simulink model "constant_f_V_PWM"  (R2016a)
settings: Solver=FixedStepAuto  StartTime=0.0  StopTime=3  FixedStep=0.00003  RelTol=1e-3
undefined symbols (not defined in the file): Lm, Lr, Ls, M_ab02abc, M_abc2ab0, Rr, sig
libraries: powerlib_meascontrol x2, simulink x1
settings Model: Creator=ebenera  LastModifiedBy=ebenera

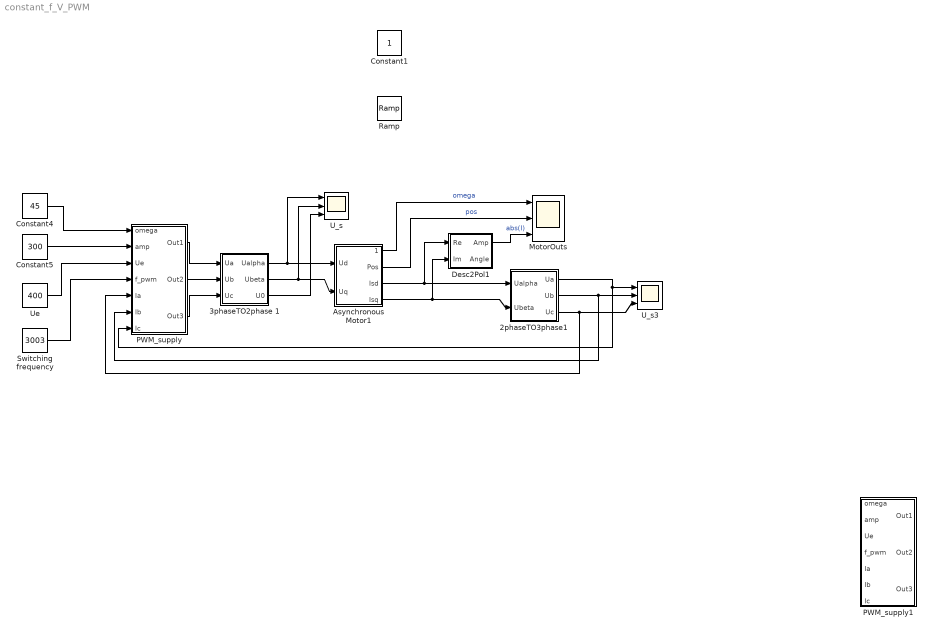
== system constant_f_V_PWM ==
  2phaseTO3phase1 : Subsystem
  3phaseTO2phase 1 : Subsystem
  Asynchronous Motor1 : Subsystem
  Constant4 : Constant  Value=45
  Constant5 : Constant  Value=300
  Desc2Pol1 : Subsystem
  MotorOuts : Scope  NumInputPorts=3
  PWM_supply : Subsystem
  PWM_supply1 : Subsystem
  Switching frequency : Constant  Value=3003
  U_s : Scope  NumInputPorts=3
  U_s3 : Scope  NumInputPorts=3
  Ue : Constant  Value=400
  " " : Constant  IOType=siggen
  Constant1 : Constant  IOType=siggen
  Ramp : simulink/Sources/Ramp  IOType=siggen  slope=1  start=0  X0=0
  wires:
  Asynchronous Motor1/4(Isq) -> 2phaseTO3phase1/2(Ubeta), Desc2Pol1/2(Im)
  Asynchronous Motor1/3(Isd) -> 2phaseTO3phase1/1(Ualpha), Desc2Pol1/1(Re)
  2phaseTO3phase1/1(Ua) -> U_s3/1, PWM_supply/7(Ic)
  2phaseTO3phase1/2(Ub) -> U_s3/2, PWM_supply/6(Ib)
  2phaseTO3phase1/3(Uc) -> U_s3/3, PWM_supply/5(Ia)
  3phaseTO2phase 1/1(Ualpha) -> U_s/1, Asynchronous Motor1/1(Ud)
  3phaseTO2phase 1/2(Ubeta) -> Asynchronous Motor1/2(Uq), U_s/2
  3phaseTO2phase 1/3(U0) -> U_s/3
  Desc2Pol1/1(Amp) -> MotorOuts/3  "abs(I)"
  Asynchronous Motor1/1(Omega) -> MotorOuts/1  "omega"
  Asynchronous Motor1/2(Pos) -> MotorOuts/2  "pos"
  Constant4/1 -> PWM_supply/1(omega)
  Constant5/1 -> PWM_supply/2(amp)
  Ue/1 -> PWM_supply/3(Ue)
  Switching frequency/1 -> PWM_supply/4(f_pwm)
  PWM_supply/1(Out1) -> 3phaseTO2phase 1/1(Ua)
  PWM_supply/2(Out2) -> 3phaseTO2phase 1/2(Ub)
  PWM_supply/3(Out3) -> 3phaseTO2phase 1/3(Uc)

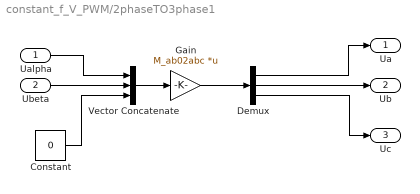
== system constant_f_V_PWM/2phaseTO3phase1 ==
  Ualpha : Inport
  Ubeta : Inport  Port=2
  Constant : Constant  Value=0
  Demux : Demux  Outputs=3
  Gain : Gain  Gain=M_ab02abc  Multiplication=Matrix(K*u)
  Vector Concatenate : Concatenate  NumInputs=3
  Ua : Outport
  Ub : Outport  Port=2
  Uc : Outport  Port=3
  wires:
  Vector Concatenate/1 -> Gain/1
  Ualpha/1 -> Vector Concatenate/1
  Demux/3 -> Uc/1
  Gain/1 -> Demux/1
  Constant/1 -> Vector Concatenate/3
  Ubeta/1 -> Vector Concatenate/2
  Demux/1 -> Ua/1
  Demux/2 -> Ub/1

== system constant_f_V_PWM/3phaseTO2phase 1 ==
  Ua : Inport
  Ub : Inport  Port=2
  Uc : Inport  Port=3
  Demux : Demux  Outputs=3
  Gain : Gain  Gain=M_abc2ab0  Multiplication=Matrix(K*u)
  Vector Concatenate : Concatenate  NumInputs=3
  Ualpha : Outport
  Ubeta : Outport  Port=2
  U0 : Outport  Port=3
  wires:
  Vector Concatenate/1 -> Gain/1
  Ua/1 -> Vector Concatenate/1
  Demux/3 -> U0/1
  Gain/1 -> Demux/1
  Uc/1 -> Vector Concatenate/3
  Ub/1 -> Vector Concatenate/2
  Demux/1 -> Ualpha/1
  Demux/2 -> Ubeta/1

== system constant_f_V_PWM/Asynchronous Motor1 ==
  Ud : Inport
  Uq : Inport  Port=2
  MeasAsync : Scope  NumInputPorts=3
  Motor Electric : Subsystem
  Motor mechanic : Subsystem
  Omega : Outport
  Pos : Outport  Port=2
  Isd : Outport  Port=3
  Isq : Outport  Port=4
  wires:
  Motor mechanic/2(Pos) -> MeasAsync/3, Pos/1  "Pos"
  Motor mechanic/1(Omega) -> Motor Electric/3(Omega), Omega/1, MeasAsync/2  "OMEGA"
  Motor Electric/1(Me) -> MeasAsync/1, Motor mechanic/1("Torq ")  "Torq"
  Motor Electric/2(Isd) -> Isd/1
  Motor Electric/3(Isq) -> Isq/1
  Uq/1 -> Motor Electric/2(Uq)
  Ud/1 -> Motor Electric/1(Ud)

== system constant_f_V_PWM/Desc2Pol1 ==
  Re : Inport
  Im : Inport  Port=2
  Complex to Magnitude-Angle2 : ComplexToMagnitudeAngle
  Real-Imag to Complex3 : RealImagToComplex
  Amp : Outport
  Angle : Outport  Port=2
  wires:
  Complex to Magnitude-Angle2/1 -> Amp/1
  Real-Imag to Complex3/1 -> Complex to Magnitude-Angle2/1
  Complex to Magnitude-Angle2/2 -> Angle/1
  Re/1 -> Real-Imag to Complex3/1
  Im/1 -> Real-Imag to Complex3/2

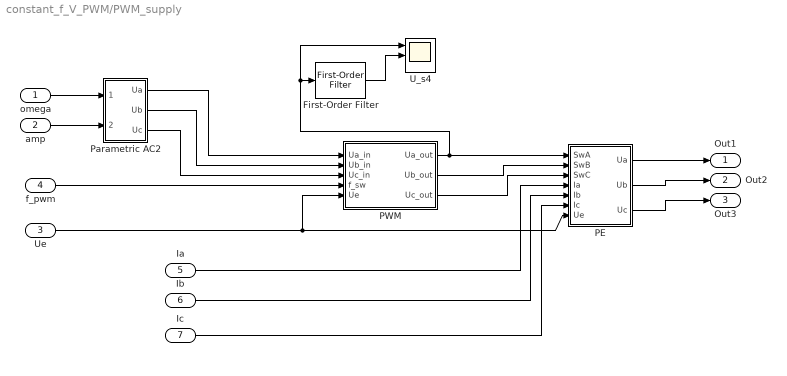
== system constant_f_V_PWM/PWM_supply ==
  omega : Inport
  amp : Inport  Port=2
  Ue : Inport  Port=3
  f_pwm : Inport  Port=4
  Ia : Inport  Port=5
  Ib : Inport  Port=6
  Ic : Inport  Port=7
  First-Order Filter : powerlib_meascontrol/Filters/First-Order Filter  FilterType=Lowpass  Tc=1/400  Ts=0  Initialize=on  Vac_Init=[0, 0, 60]  Vdc_Init=0  PlotResponse=off  FreqRange="[0,  200,  1]"
  PE : Subsystem
  PWM : Subsystem
  Parametric AC2 : Subsystem  Description=Generates a 3 phase supply with the given angular speed, and aplitude.
  U_s4 : Scope  NumInputPorts=3
  Out1 : Outport
  Out2 : Outport  Port=2
  Out3 : Outport  Port=3
  wires:
  Ic/1 -> PE/6(Ic)
  Ia/1 -> PE/4(Ia)
  Ib/1 -> PE/5(Ib)
  Parametric AC2/3(Uc) -> PWM/3(Uc_in)
  f_pwm/1 -> PWM/4(f_sw)
  Parametric AC2/2(Ub) -> PWM/2(Ub_in)
  amp/1 -> Parametric AC2/2(Amp)
  First-Order Filter/1 -> U_s4/2
  PWM/2(Ub_out) -> PE/2(SwB)
  PWM/1(Ua_out) -> PE/1(SwA), U_s4/1, First-Order Filter/1
  PWM/3(Uc_out) -> PE/3(SwC)
  omega/1 -> Parametric AC2/1(Omega)
  Parametric AC2/1(Ua) -> PWM/1(Ua_in)
  PE/1(Ua) -> Out1/1
  PE/2(Ub) -> Out2/1
  PE/3(Uc) -> Out3/1
  Ue/1 -> PE/7(Ue), PWM/5(Ue)

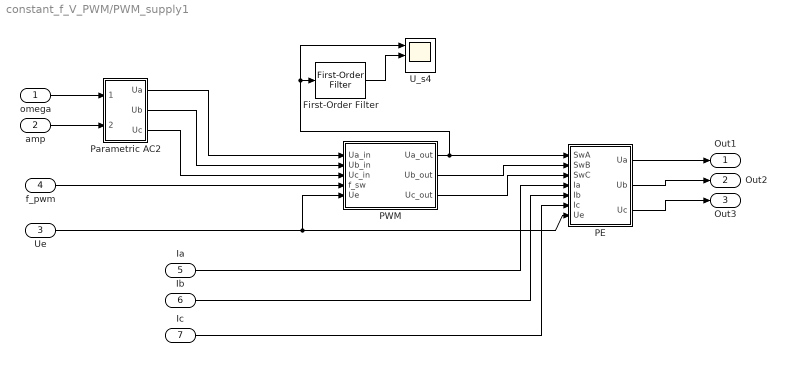
== system constant_f_V_PWM/PWM_supply1 ==
  omega : Inport
  amp : Inport  Port=2
  Ue : Inport  Port=3
  f_pwm : Inport  Port=4
  Ia : Inport  Port=5
  Ib : Inport  Port=6
  Ic : Inport  Port=7
  First-Order Filter : powerlib_meascontrol/Filters/First-Order Filter  FilterType=Lowpass  Tc=1/400  Ts=0  Initialize=on  Vac_Init=[0, 0, 60]  Vdc_Init=0  PlotResponse=off  FreqRange="[0,  200,  1]"
  PE : Subsystem
  PWM : Subsystem
  Parametric AC2 : Subsystem  Description=Generates a 3 phase supply with the given angular speed, and aplitude.
  U_s4 : Scope  NumInputPorts=3
  Out1 : Outport
  Out2 : Outport  Port=2
  Out3 : Outport  Port=3
  wires:
  Ic/1 -> PE/6(Ic)
  Ia/1 -> PE/4(Ia)
  Ib/1 -> PE/5(Ib)
  Parametric AC2/3(Uc) -> PWM/3(Uc_in)
  f_pwm/1 -> PWM/4(f_sw)
  Parametric AC2/2(Ub) -> PWM/2(Ub_in)
  amp/1 -> Parametric AC2/2(Amp)
  First-Order Filter/1 -> U_s4/2
  PWM/2(Ub_out) -> PE/2(SwB)
  PWM/1(Ua_out) -> PE/1(SwA), U_s4/1, First-Order Filter/1
  PWM/3(Uc_out) -> PE/3(SwC)
  omega/1 -> Parametric AC2/1(Omega)
  Parametric AC2/1(Ua) -> PWM/1(Ua_in)
  PE/1(Ua) -> Out1/1
  PE/2(Ub) -> Out2/1
  PE/3(Uc) -> Out3/1
  Ue/1 -> PE/7(Ue), PWM/5(Ue)

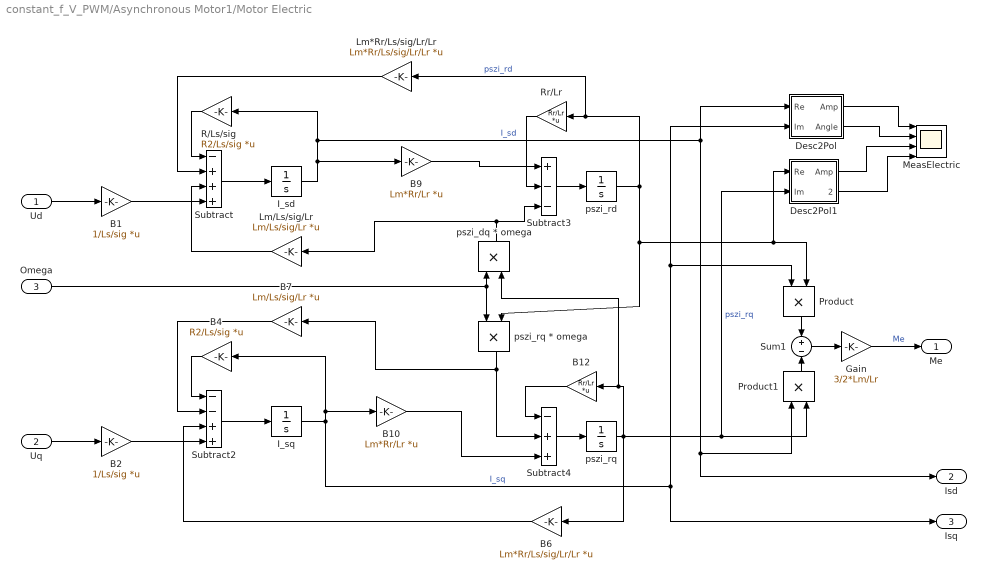
== system constant_f_V_PWM/Asynchronous Motor1/Motor Electric ==
  Ud : Inport
  Uq : Inport  Port=2
  Omega : Inport  Port=3
  B1 : Gain  Gain=1/Ls/sig  Multiplication=Matrix(K*u)
  B10 : Gain  Gain=Lm*Rr/Lr  Multiplication=Matrix(K*u)
  B12 : Gain  Gain=Rr/Lr  Multiplication=Matrix(K*u)
  B2 : Gain  Gain=1/Ls/sig  Multiplication=Matrix(K*u)
  B4 : Gain  Gain=R2/Ls/sig  Multiplication=Matrix(K*u)
  B6 : Gain  Gain=Lm*Rr/Ls/sig/Lr/Lr  Multiplication=Matrix(K*u)
  B7 : Gain  Gain=Lm/Ls/sig/Lr  Multiplication=Matrix(K*u)
  B9 : Gain  Gain=Lm*Rr/Lr  Multiplication=Matrix(K*u)
  Desc2Pol : Subsystem
  Desc2Pol1 : Subsystem
  Gain : Gain  Gain=3/2*Lm/Lr
  I_sd : Integrator
  I_sq : Integrator
  Lm*Rr/Ls/sig/Lr/Lr : Gain  Gain=Lm*Rr/Ls/sig/Lr/Lr  Multiplication=Matrix(K*u)
  Lm/Ls/sig/Lr : Gain  Gain=Lm/Ls/sig/Lr  Multiplication=Matrix(K*u)
  MeasElectric : Scope  NumInputPorts=4
  Product : Product
  Product1 : Product
  R/Ls/sig : Gain  Gain=R2/Ls/sig  Multiplication=Matrix(K*u)
  Rr/Lr : Gain  Gain=Rr/Lr  Multiplication=Matrix(K*u)
  Subtract : Sum  Inputs=-+++
  Subtract2 : Sum  Inputs=--++
  Subtract3 : Sum  Inputs=+--
  Subtract4 : Sum  Inputs=-++
  Sum1 : Sum  Inputs=+-
  pszi_dq * omega : Product
  pszi_rd : Integrator
  "pszi_rq " : Integrator
  pszi_rq * omega : Product
  Me : Outport
  Isd : Outport  Port=2
  Isq : Outport  Port=3
  wires:
  pszi_rq * omega/1 -> Subtract4/2, B7/1
  Subtract/1 -> I_sd/1
  B12/1 -> Subtract4/1
  Product1/1 -> Sum1/2
  Lm*Rr/Ls/sig/Lr/Lr/1 -> Subtract/2
  Product/1 -> Sum1/1
  I_sq/1 -> Product/1, Desc2Pol/2(Im), Isq/1, B10/1, B4/1  "I_sq"
  I_sd/1 -> B9/1, Isd/1, Product1/1, Desc2Pol/1(Re), R/Ls/sig/1  "I_sd"
  Sum1/1 -> Gain/1
  R/Ls/sig/1 -> Subtract/1
  B6/1 -> Subtract2/3
  B4/1 -> Subtract2/1
  pszi_dq * omega/1 -> Subtract3/3, Lm/Ls/sig/Lr/1
  Omega/1 -> pszi_rq * omega/1, pszi_dq * omega/1
  B9/1 -> Subtract3/1
  Rr/Lr/1 -> Subtract3/2
  pszi_rd/1 -> Product/2, Desc2Pol1/1(Re), pszi_rq * omega/2, Lm*Rr/Ls/sig/Lr/Lr/1, Rr/Lr/1  "pszi_rd"
  Lm/Ls/sig/Lr/1 -> Subtract/3
  "pszi_rq "/1 -> B6/1, Product1/2, Desc2Pol1/2(Im), pszi_dq * omega/2, B12/1  "pszi_rq"
  B7/1 -> Subtract2/2
  Gain/1 -> Me/1  "Me"
  B10/1 -> Subtract4/3
  Subtract4/1 -> "pszi_rq "/1
  Subtract2/1 -> I_sq/1
  Subtract3/1 -> pszi_rd/1
  Uq/1 -> B2/1
  Ud/1 -> B1/1
  B1/1 -> Subtract/4
  B2/1 -> Subtract2/4
  Desc2Pol/1(Amp) -> MeasElectric/1
  Desc2Pol/2(Angle) -> MeasElectric/2
  Desc2Pol1/1(Amp) -> MeasElectric/3
  Desc2Pol1/2(Angle) -> MeasElectric/4

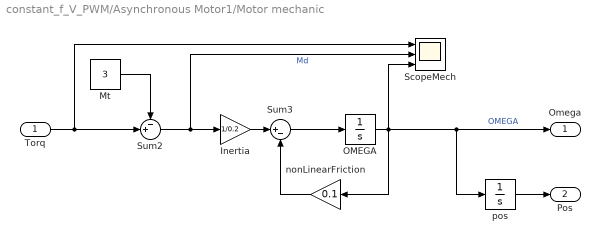
== system constant_f_V_PWM/Asynchronous Motor1/Motor mechanic ==
  "Torq " : Inport
  Inertia : Gain  Gain=1/0.2
  Mt : Constant  Value=3
  OMEGA : Integrator
  ScopeMech : Scope  NumInputPorts=3
  Sum2 : Sum  Inputs=-+|
  Sum3 : Sum  Inputs=|+-
  nonLinearFriction : Gain  Gain=0.1
  pos : Integrator  WrapState=on
  Omega : Outport
  Pos : Outport  Port=2
  wires:
  "Torq "/1 -> ScopeMech/1, Sum2/2
  OMEGA/1 -> ScopeMech/3, pos/1, Omega/1, nonLinearFriction/1  "OMEGA"
  Sum3/1 -> OMEGA/1
  Sum2/1 -> Inertia/1, ScopeMech/2  "Md"
  Mt/1 -> Sum2/1
  nonLinearFriction/1 -> Sum3/2
  Inertia/1 -> Sum3/1
  pos/1 -> Pos/1

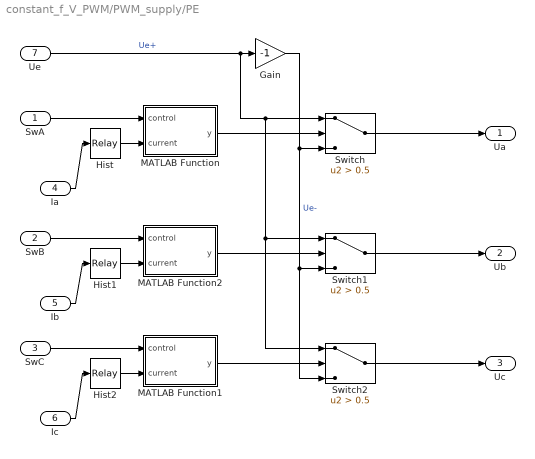
== system constant_f_V_PWM/PWM_supply/PE ==
  SwA : Inport
  SwB : Inport  Port=2
  SwC : Inport  Port=3
  Ia : Inport  Port=4
  Ib : Inport  Port=5
  Ic : Inport  Port=6
  Ue : Inport  Port=7
  Gain : Gain  Gain=-1
  Hist : Relay  OnSwitchValue=0.1  OffSwitchValue=-0.1  OffOutputValue=-1
  Hist1 : Relay  OnSwitchValue=0.1  OffSwitchValue=-0.1  OffOutputValue=-1
  Hist2 : Relay  OnSwitchValue=0.1  OffSwitchValue=-0.1  OffOutputValue=-1
  MATLAB Function : MATLAB Function  TreatAsAtomicUnit=on
  MATLAB Function1 : MATLAB Function  TreatAsAtomicUnit=on
  MATLAB Function2 : MATLAB Function  TreatAsAtomicUnit=on
  Switch : Switch  Criteria=u2 > Threshold  Threshold=0.5
  Switch1 : Switch  Criteria=u2 > Threshold  Threshold=0.5
  Switch2 : Switch  Criteria=u2 > Threshold  Threshold=0.5
  Ua : Outport
  Ub : Outport  Port=2
  Uc : Outport  Port=3
  wires:
  Gain/1 -> Switch2/3, Switch1/3, Switch/3  "Ue-"
  Switch/1 -> Ua/1
  Ue/1 -> Switch/1, Switch1/1, Switch2/1, Gain/1  "Ue+"
  Switch1/1 -> Ub/1
  Switch2/1 -> Uc/1
  MATLAB Function/1(y) -> Switch/2
  MATLAB Function2/1(y) -> Switch1/2
  MATLAB Function1/1(y) -> Switch2/2
  SwB/1 -> MATLAB Function2/1(control)
  SwA/1 -> MATLAB Function/1(control)
  SwC/1 -> MATLAB Function1/1(control)
  Ia/1 -> Hist/1
  Hist/1 -> MATLAB Function/2(current)
  Ib/1 -> Hist1/1
  Hist1/1 -> MATLAB Function2/2(current)
  Hist2/1 -> MATLAB Function1/2(current)
  Ic/1 -> Hist2/1

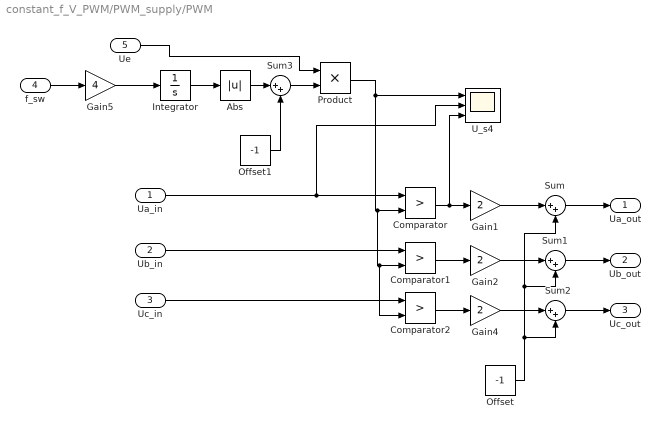
== system constant_f_V_PWM/PWM_supply/PWM ==
  Ua_in : Inport
  Ub_in : Inport  Port=2
  Uc_in : Inport  Port=3
  f_sw : Inport  Port=4
  Ue : Inport  Port=5
  Abs : Abs
  Comparator : RelationalOperator  Operator=>  OutDataTypeStr=boolean
  Comparator1 : RelationalOperator  Operator=>  OutDataTypeStr=boolean
  Comparator2 : RelationalOperator  Operator=>  OutDataTypeStr=boolean
  Gain1 : Gain  Gain=2
  Gain2 : Gain  Gain=2
  Gain4 : Gain  Gain=2
  Gain5 : Gain  Gain=4
  Integrator : Integrator  WrapState=on  WrappedStateUpperValue=2  WrappedStateLowerValue=-2
  Offset : Constant  Value=-1
  Offset1 : Constant  Value=-1
  Product : Product
  Sum{,1..3} (4 alike) : Sum  Inputs=|++
  U_s4 : Scope  NumInputPorts=3
  Ua_out : Outport
  Ub_out : Outport  Port=2
  Uc_out : Outport  Port=3
  wires:
  Uc_in/1 -> Comparator2/1
  Ub_in/1 -> Comparator1/1
  Ua_in/1 -> U_s4/2, Comparator/1
  Comparator/1 -> Gain1/1, U_s4/3
  Product/1 -> U_s4/1, Comparator2/2, Comparator1/2, Comparator/2
  Gain2/1 -> Sum1/1
  Comparator1/1 -> Gain2/1
  Comparator2/1 -> Gain4/1
  Gain4/1 -> Sum2/1
  Sum2/1 -> Uc_out/1
  Sum1/1 -> Ub_out/1
  Sum/1 -> Ua_out/1
  Gain1/1 -> Sum/1
  Offset/1 -> Sum2/2, Sum1/2, Sum/2
  Gain5/1 -> Integrator/1
  f_sw/1 -> Gain5/1
  Ue/1 -> Product/1
  Integrator/1 -> Abs/1
  Offset1/1 -> Sum3/2
  Abs/1 -> Sum3/1
  Sum3/1 -> Product/2

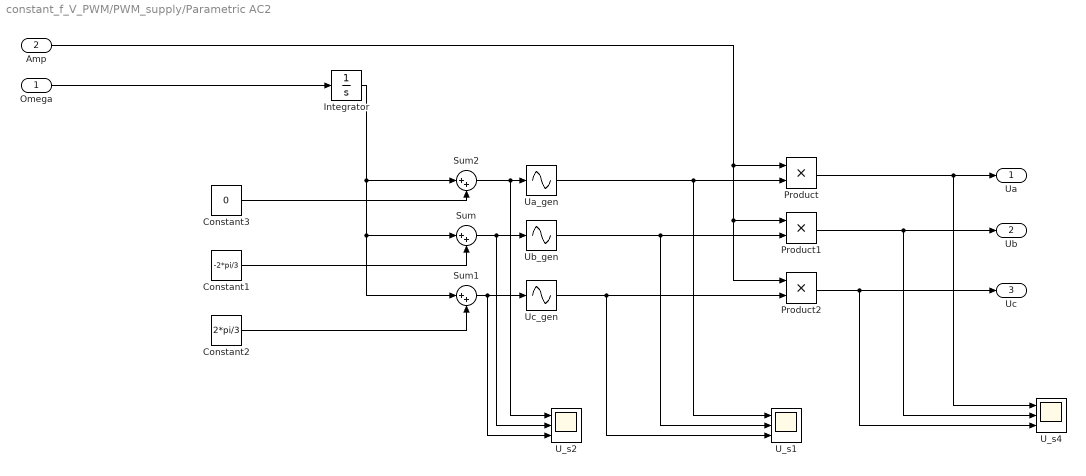
== system constant_f_V_PWM/PWM_supply/Parametric AC2 ==
  Omega : Inport
  Amp : Inport  Port=2
  Constant1 : Constant  Value=-2*pi/3
  Constant2 : Constant  Value=2*pi/3
  Constant3 : Constant  Value=0
  Integrator : Integrator  WrapState=on
  Product : Product
  Product1 : Product
  Product2 : Product
  Sum : Sum  Inputs=|++
  Sum1 : Sum  Inputs=|++
  Sum2 : Sum  Inputs=|++
  U_s1 : Scope  NumInputPorts=3
  U_s2 : Scope  NumInputPorts=3
  U_s4 : Scope  NumInputPorts=3
  Ua_gen : Sin  TimeSource=Use external signal  SampleTime=0
  Ub_gen : Sin  TimeSource=Use external signal  SampleTime=0
  Uc_gen : Sin  TimeSource=Use external signal  SampleTime=0
  Ua : Outport
  Ub : Outport  Port=2
  Uc : Outport  Port=3
  wires:
  Sum/1 -> U_s2/2, Ub_gen/1
  Omega/1 -> Integrator/1
  Constant1/1 -> Sum/2
  Constant2/1 -> Sum1/2
  Sum1/1 -> U_s2/3, Uc_gen/1
  Sum2/1 -> U_s2/1, Ua_gen/1
  Constant3/1 -> Sum2/2
  Integrator/1 -> Sum2/1, Sum1/1, Sum/1
  Product/1 -> U_s4/1, Ua/1
  Product2/1 -> U_s4/3, Uc/1
  Product1/1 -> U_s4/2, Ub/1
  Amp/1 -> Product/1, Product1/1, Product2/1
  Ua_gen/1 -> U_s1/1, Product/2
  Uc_gen/1 -> U_s1/3, Product2/2
  Ub_gen/1 -> U_s1/2, Product1/2

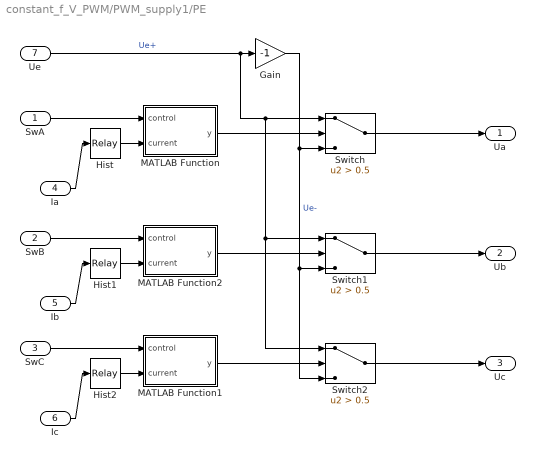
== system constant_f_V_PWM/PWM_supply1/PE ==
  SwA : Inport
  SwB : Inport  Port=2
  SwC : Inport  Port=3
  Ia : Inport  Port=4
  Ib : Inport  Port=5
  Ic : Inport  Port=6
  Ue : Inport  Port=7
  Gain : Gain  Gain=-1
  Hist : Relay  OnSwitchValue=0.1  OffSwitchValue=-0.1  OffOutputValue=-1
  Hist1 : Relay  OnSwitchValue=0.1  OffSwitchValue=-0.1  OffOutputValue=-1
  Hist2 : Relay  OnSwitchValue=0.1  OffSwitchValue=-0.1  OffOutputValue=-1
  MATLAB Function : MATLAB Function  TreatAsAtomicUnit=on
  MATLAB Function1 : MATLAB Function  TreatAsAtomicUnit=on
  MATLAB Function2 : MATLAB Function  TreatAsAtomicUnit=on
  Switch : Switch  Criteria=u2 > Threshold  Threshold=0.5
  Switch1 : Switch  Criteria=u2 > Threshold  Threshold=0.5
  Switch2 : Switch  Criteria=u2 > Threshold  Threshold=0.5
  Ua : Outport
  Ub : Outport  Port=2
  Uc : Outport  Port=3
  wires:
  Gain/1 -> Switch2/3, Switch1/3, Switch/3  "Ue-"
  Switch/1 -> Ua/1
  Ue/1 -> Switch/1, Switch1/1, Switch2/1, Gain/1  "Ue+"
  Switch1/1 -> Ub/1
  Switch2/1 -> Uc/1
  MATLAB Function/1(y) -> Switch/2
  MATLAB Function2/1(y) -> Switch1/2
  MATLAB Function1/1(y) -> Switch2/2
  SwB/1 -> MATLAB Function2/1(control)
  SwA/1 -> MATLAB Function/1(control)
  SwC/1 -> MATLAB Function1/1(control)
  Ia/1 -> Hist/1
  Hist/1 -> MATLAB Function/2(current)
  Ib/1 -> Hist1/1
  Hist1/1 -> MATLAB Function2/2(current)
  Hist2/1 -> MATLAB Function1/2(current)
  Ic/1 -> Hist2/1

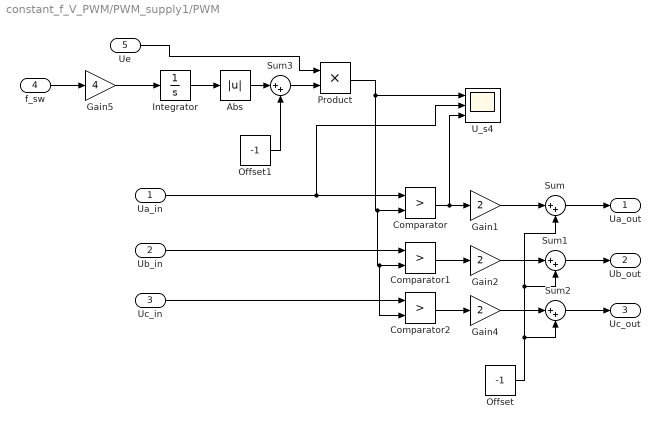
== system constant_f_V_PWM/PWM_supply1/PWM ==
  Ua_in : Inport
  Ub_in : Inport  Port=2
  Uc_in : Inport  Port=3
  f_sw : Inport  Port=4
  Ue : Inport  Port=5
  Abs : Abs
  Comparator : RelationalOperator  Operator=>  OutDataTypeStr=boolean
  Comparator1 : RelationalOperator  Operator=>  OutDataTypeStr=boolean
  Comparator2 : RelationalOperator  Operator=>  OutDataTypeStr=boolean
  Gain1 : Gain  Gain=2
  Gain2 : Gain  Gain=2
  Gain4 : Gain  Gain=2
  Gain5 : Gain  Gain=4
  Integrator : Integrator  WrapState=on  WrappedStateUpperValue=2  WrappedStateLowerValue=-2
  Offset : Constant  Value=-1
  Offset1 : Constant  Value=-1
  Product : Product
  Sum{,1..3} (4 alike) : Sum  Inputs=|++
  U_s4 : Scope  NumInputPorts=3
  Ua_out : Outport
  Ub_out : Outport  Port=2
  Uc_out : Outport  Port=3
  wires:
  Uc_in/1 -> Comparator2/1
  Ub_in/1 -> Comparator1/1
  Ua_in/1 -> U_s4/2, Comparator/1
  Comparator/1 -> Gain1/1, U_s4/3
  Product/1 -> U_s4/1, Comparator2/2, Comparator1/2, Comparator/2
  Gain2/1 -> Sum1/1
  Comparator1/1 -> Gain2/1
  Comparator2/1 -> Gain4/1
  Gain4/1 -> Sum2/1
  Sum2/1 -> Uc_out/1
  Sum1/1 -> Ub_out/1
  Sum/1 -> Ua_out/1
  Gain1/1 -> Sum/1
  Offset/1 -> Sum2/2, Sum1/2, Sum/2
  Gain5/1 -> Integrator/1
  f_sw/1 -> Gain5/1
  Ue/1 -> Product/1
  Integrator/1 -> Abs/1
  Offset1/1 -> Sum3/2
  Abs/1 -> Sum3/1
  Sum3/1 -> Product/2

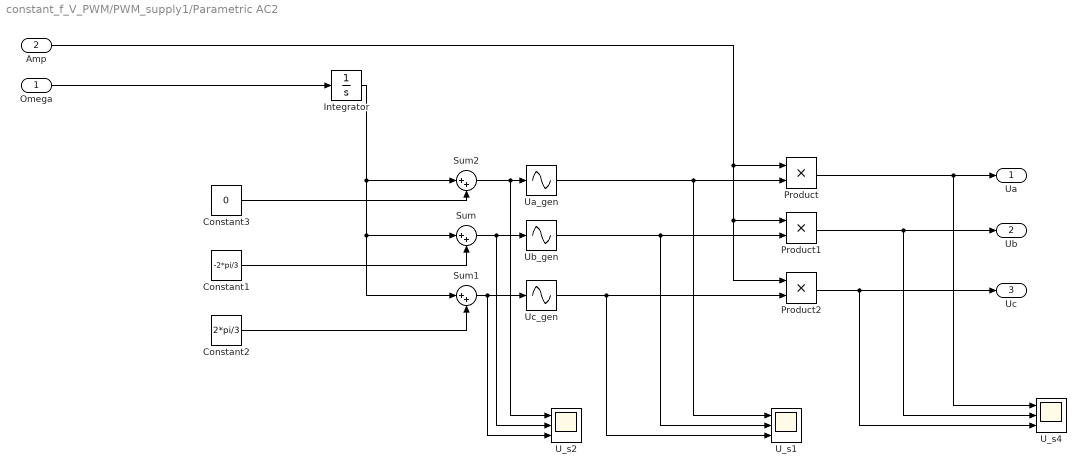
== system constant_f_V_PWM/PWM_supply1/Parametric AC2 ==
  Omega : Inport
  Amp : Inport  Port=2
  Constant1 : Constant  Value=-2*pi/3
  Constant2 : Constant  Value=2*pi/3
  Constant3 : Constant  Value=0
  Integrator : Integrator  WrapState=on
  Product : Product
  Product1 : Product
  Product2 : Product
  Sum : Sum  Inputs=|++
  Sum1 : Sum  Inputs=|++
  Sum2 : Sum  Inputs=|++
  U_s1 : Scope  NumInputPorts=3
  U_s2 : Scope  NumInputPorts=3
  U_s4 : Scope  NumInputPorts=3
  Ua_gen : Sin  TimeSource=Use external signal  SampleTime=0
  Ub_gen : Sin  TimeSource=Use external signal  SampleTime=0
  Uc_gen : Sin  TimeSource=Use external signal  SampleTime=0
  Ua : Outport
  Ub : Outport  Port=2
  Uc : Outport  Port=3
  wires:
  Sum/1 -> U_s2/2, Ub_gen/1
  Omega/1 -> Integrator/1
  Constant1/1 -> Sum/2
  Constant2/1 -> Sum1/2
  Sum1/1 -> U_s2/3, Uc_gen/1
  Sum2/1 -> U_s2/1, Ua_gen/1
  Constant3/1 -> Sum2/2
  Integrator/1 -> Sum2/1, Sum1/1, Sum/1
  Product/1 -> U_s4/1, Ua/1
  Product2/1 -> U_s4/3, Uc/1
  Product1/1 -> U_s4/2, Ub/1
  Amp/1 -> Product/1, Product1/1, Product2/1
  Ua_gen/1 -> U_s1/1, Product/2
  Uc_gen/1 -> U_s1/3, Product2/2
  Ub_gen/1 -> U_s1/2, Product1/2

== system constant_f_V_PWM/Asynchronous Motor1/Motor Electric/Desc2Pol ==
  Re : Inport
  Im : Inport  Port=2
  Complex to Magnitude-Angle2 : ComplexToMagnitudeAngle
  Real-Imag to Complex3 : RealImagToComplex
  Amp : Outport
  Angle : Outport  Port=2
  wires:
  Complex to Magnitude-Angle2/1 -> Amp/1
  Real-Imag to Complex3/1 -> Complex to Magnitude-Angle2/1
  Complex to Magnitude-Angle2/2 -> Angle/1
  Re/1 -> Real-Imag to Complex3/1
  Im/1 -> Real-Imag to Complex3/2

== system constant_f_V_PWM/Asynchronous Motor1/Motor Electric/Desc2Pol1 ==
  Re : Inport
  Im : Inport  Port=2
  Complex to Magnitude-Angle2 : ComplexToMagnitudeAngle
  Real-Imag to Complex3 : RealImagToComplex
  Amp : Outport
  Angle : Outport  Port=2
  wires:
  Complex to Magnitude-Angle2/1 -> Amp/1
  Real-Imag to Complex3/1 -> Complex to Magnitude-Angle2/1
  Complex to Magnitude-Angle2/2 -> Angle/1
  Re/1 -> Real-Imag to Complex3/1
  Im/1 -> Real-Imag to Complex3/2

== matlab function constant_f_V_PWM/PWM_supply/PE/MATLAB Function1 ==
  data: control input; y output; current input
function y = fcn(control, current)
	if control >= 1
        y = 1;
    elseif control <= -1
        y=-1;
    elseif(current>0)
        y = -1;
    else
        y = 1;
    end
end

== matlab function constant_f_V_PWM/PWM_supply/PE/MATLAB Function ==
  data: control input; y output; current input
function y = fcn(control, current)
	if control > 0.5
        y = 1;
    elseif control < -0.5
        y=-1;
    elseif(current>0)
        y = -1;
    else
        y = 1;
    end
end

== matlab function constant_f_V_PWM/PWM_supply/PE/MATLAB Function2 ==
  data: control input; y output; current input
function y = fcn(control, current)
	if control >= 1
        y = 1;
    elseif control <= -1
        y=-1;
    elseif(current>0)
        y = -1;
    else
        y = 1;
    end
end

== matlab function constant_f_V_PWM/PWM_supply1/PE/MATLAB Function ==
  data: control input; y output; current input
function y = fcn(control, current)
	if control > 0.5
        y = 1;
    elseif control < -0.5
        y=-1;
    elseif(current>0)
        y = -1;
    else
        y = 1;
    end
end

== matlab function constant_f_V_PWM/PWM_supply1/PE/MATLAB Function1 ==
  data: control input; y output; current input
function y = fcn(control, current)
	if control >= 1
        y = 1;
    elseif control <= -1
        y=-1;
    elseif(current>0)
        y = -1;
    else
        y = 1;
    end
end

== matlab function constant_f_V_PWM/PWM_supply1/PE/MATLAB Function2 ==
  data: control input; y output; current input
function y = fcn(control, current)
	if control >= 1
        y = 1;
    elseif control <= -1
        y=-1;
    elseif(current>0)
        y = -1;
    else
        y = 1;
    end
end
